simulink model "RLC_Circuit"  (R2022b)
settings: Solver=FixedStepAuto  StartTime=0.0  StopTime=10.0  FixedStep=1e-3  RelTol=1e-3
settings Model: Creator=yasso  LastModifiedBy=yasso

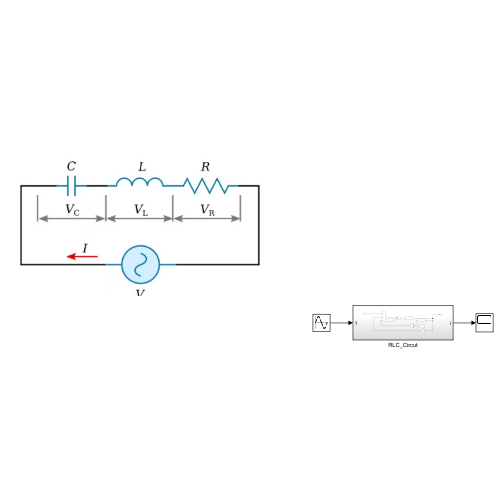
[thumbnail: Simulink's stored preview of the top-level diagram]
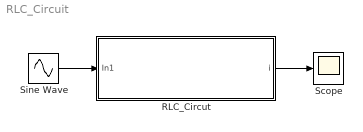
== system RLC_Circuit ==
  RLC_Circut : Subsystem
  Scope : Scope
  Sine Wave : Sin  SampleTime=0
  wires:
  Sine Wave/1 -> RLC_Circut/1(In1)
  RLC_Circut/1(i) -> Scope/1

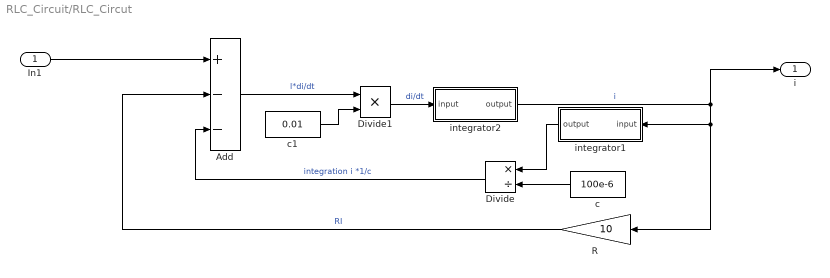
== system RLC_Circuit/RLC_Circut ==
  In1 : Inport
  Add : Sum  Inputs=+--
  Divide : Product  Inputs=*/
  Divide1 : Product  Inputs=**
  R : Gain  Gain=10
  c : Constant  Value=100e-6
  c1 : Constant  Value=0.01
  integrator1 : Subsystem
  integrator2 : Subsystem
  i : Outport
  wires:
  In1/1 -> Add/1
  Divide1/1 -> integrator2/1(input)  "di/dt"
  integrator1/1(output) -> Divide/1
  R/1 -> Add/2  "RI"
  c/1 -> Divide/2
  Add/1 -> Divide1/1  "l*di/dt"
  Divide/1 -> Add/3  "integration i *1/c"
  c1/1 -> Divide1/2
  integrator2/1(output) -> i/1, integrator1/1(input), R/1  "i"

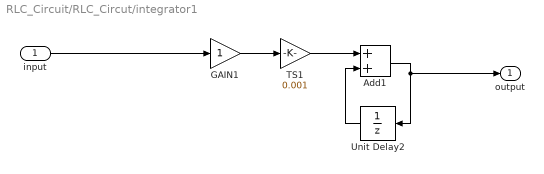
== system RLC_Circuit/RLC_Circut/integrator1 ==
  input : Inport
  Add1 : Sum
  GAIN1 : Gain
  TS1 : Gain  Gain=0.001
  Unit Delay2 : UnitDelay  SampleTime=-1  HasFrameUpgradeWarning=on
  output : Outport
  wires:
  Unit Delay2/1 -> Add1/2
  TS1/1 -> Add1/1
  input/1 -> GAIN1/1
  Add1/1 -> Unit Delay2/1, output/1
  GAIN1/1 -> TS1/1

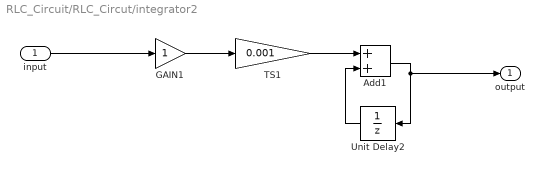
== system RLC_Circuit/RLC_Circut/integrator2 ==
  input : Inport
  Add1 : Sum
  GAIN1 : Gain
  TS1 : Gain  Gain=0.001
  Unit Delay2 : UnitDelay  SampleTime=-1  HasFrameUpgradeWarning=on
  output : Outport
  wires:
  GAIN1/1 -> TS1/1
  Add1/1 -> output/1, Unit Delay2/1
  input/1 -> GAIN1/1
  TS1/1 -> Add1/1
  Unit Delay2/1 -> Add1/2
